simulink model "untitled"  (R2024b)
settings: Solver=VariableStepAuto  StartTime=0.0  StopTime=10.0  RelTol=1e-3
libraries: spspowerguiLib x1
settings Model: Creator=G5  LastModifiedBy=G5

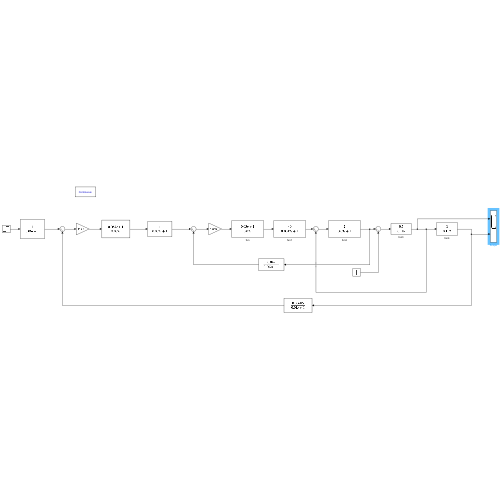
[thumbnail: Simulink's stored preview of the top-level diagram]
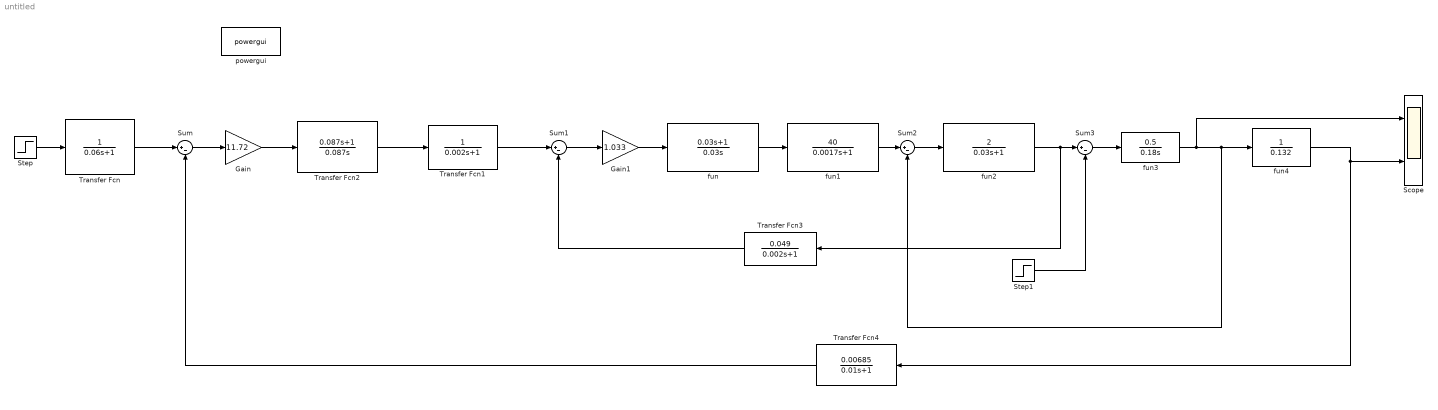
== system untitled ==
  Gain : Gain  Gain=11.72
  Gain1 : Gain  Gain=1.033
  Scope : Scope  NumInputPorts=2
  Step : Step  Time=0  After=10  SampleTime=0
  Step1 : Step  Time=0  After=10  SampleTime=0
  Sum{,1..3} (4 alike) : Sum  Inputs=|+-
  Transfer Fcn : TransferFcn  Denominator=[0.06 1]
  Transfer Fcn1 : TransferFcn  Denominator=[0.002 1]
  Transfer Fcn2 : TransferFcn  Numerator=[0.087 1]  Denominator=[0.087 0]
  Transfer Fcn3 : TransferFcn  Numerator=[0.049]  Denominator=[0.002 1]
  Transfer Fcn4 : TransferFcn  Numerator=[0.00685]  Denominator=[0.01 1]
  fun : TransferFcn  Numerator=[0.03 1]  Denominator=[0.03 0]
  fun1 : TransferFcn  Numerator=[40]  Denominator=[0.0017 1]
  fun2 : TransferFcn  Numerator=[2]  Denominator=[0.03 1]
  fun3 : TransferFcn  Numerator=[0.5]  Denominator=[0.18 0]
  fun4 : TransferFcn  Denominator=[0.132]
  powergui : spspowerguiLib/powergui  Priority=1  SimulationMode=Continuous  SampleTime=50e-6  frequency=60  Iterations=50  frequencyindice=60  Pbase=100e6  ErrMax=1e-4  UnitsV=kV  UnitsW=MW  buscounter=0  FunctionMessages=off  echomessages=off  EnableUseOfTLC=off  CurrentSourceSwitches=off  DisableSnubberDevices=off  DisableRonSwitches=off  DisableVfSwitches=off  DisplayEquations=off  AutomaticDiscreteSolvers=off  SolverType=Tustin/Backward Euler (TBE)  Interpol=off  ExternalGateDelay=off  methode=off  Ts=100  x0status=blocks  SPID=on  SwTol=0  HookPort=off  NonlinearTolerance=1e-4  nMaxIteration=100  ContinueOnMaxIteration=off  RestoreLinks=warning  ResistiveCurrentMeasurement=off  Frange=[0:2:500]  Ylog=off  Xlog=on  ShowGrid=off  save=off  variable=ZData  structure=0  ZoomFFT=off  StartTime=0.0  cycles=1  DisplayStyle=1  fundamental=60  FreqAxis=off  MaxFrequency=1000  frequencyindicesteady=1  RmsSteady=1  display=off
  wires:
  Step/1 -> Transfer Fcn/1
  Transfer Fcn4/1 -> Sum/2
  fun2/1 -> Transfer Fcn3/1, Sum3/1
  Gain1/1 -> fun/1
  Sum/1 -> Gain/1
  Gain/1 -> Transfer Fcn2/1
  Transfer Fcn/1 -> Sum/1
  Step1/1 -> Sum3/2
  fun4/1 -> Transfer Fcn4/1, Scope/2
  Sum2/1 -> fun2/1
  Transfer Fcn3/1 -> Sum1/2
  Transfer Fcn2/1 -> Transfer Fcn1/1
  Sum1/1 -> Gain1/1
  fun3/1 -> Scope/1, Sum2/2, fun4/1
  Sum3/1 -> fun3/1
  fun/1 -> fun1/1
  fun1/1 -> Sum2/1
  Transfer Fcn1/1 -> Sum1/1
